simulink model "feedbacklin"  (R2020b)
settings: Solver=VariableStepAuto  StartTime=0.0  StopTime=40  RelTol=1e-3
values from neighbouring files (symbols this model uses):
  Ax = 25    [main.m]
  Ay = 25    [main.m]
  d2x = sym('d2x', 'real')    [AL.m]    (also in FL.m; main.m = 0)
  d2z = sym('d2z', 'real')    [AL.m]    (also in FL.m; main.m = 0.0979)
  dgx = sym('dgx', 'real')    [AL.m]    (also in FL.m; main.m = 0)
  gravity = sym('gravity','real')    [AL.m]    (also in FL.m; main.m = 9.81)
  J1 = sym('J1', 'real')    [AL.m]    (also in FL.m; main.m = 0.0154)
  J2 = sym('J2', 'real')    [AL.m]    (also in FL.m; main.m = 0.0011)
  Jm = sym('Jm', 'real')    [AL.m]    (also in FL.m; main.m = 0.4101)
  m1 = sym('m1','real')    [AL.m]    (also in FL.m; main.m = 1.309)
  m2 = sym('m2','real')    [AL.m]    (also in FL.m; main.m = 0.098)
  mM = sym('mM','real')    [AL.m]    (also in FL.m = sym('m','real'); main.m = 0.06)
  selector = select(1)    [main.m]    (also in select.m = input('? '))
  wx = 0.16    [main.m]
  wy = 0.16    [main.m]
(part 1 of 2)
settings Model: Creator=Tommaso  LastModifiedBy=Tommaso
settings DataIOCC: ReturnWorkspaceOutputs=off

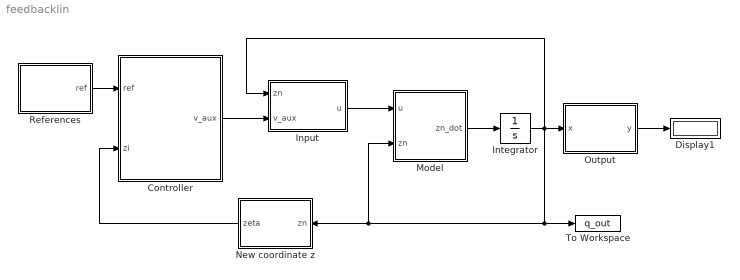
== system feedbacklin ==
  Controller : MATLAB Function  TreatAsAtomicUnit=on
  Display1 : Display
  Input : MATLAB Function  TreatAsAtomicUnit=on
  Integrator : Integrator  InitialCondition=[0; 0; 0; 0; 0; 0; 0; 0; (m1+m2+mM)*gravity; 0; 0; 0]
  Model : MATLAB Function  TreatAsAtomicUnit=on
  New coordinate z : MATLAB Function  TreatAsAtomicUnit=on
  Output : MATLAB Function  TreatAsAtomicUnit=on
  References : Subsystem
  To Workspace : ToWorkspace  VariableName=q_out  SaveFormat=Timeseries  SampleTime=-1
  wires:
  Output/1(y) -> Display1/1
  Integrator/1 -> Output/1(x), To Workspace/1, Model/2(zn), New coordinate z/1(zn), Input/1(zn)
  Model/1(zn_dot) -> Integrator/1
  Input/1(u) -> Model/1(u)
  Controller/1(v_aux) -> Input/2(v_aux)
  New coordinate z/1(zeta) -> Controller/2(zi)
  References/1(ref) -> Controller/1(ref)

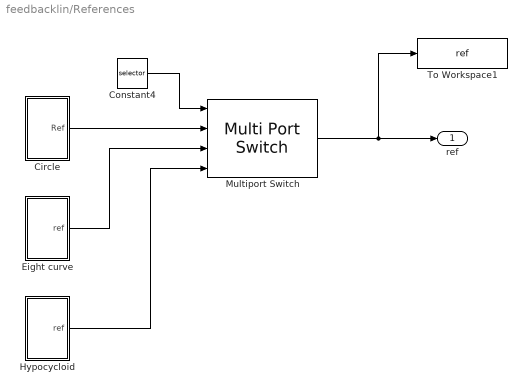
== system feedbacklin/References ==
  Circle : Subsystem
  Constant4 : Constant  Value=selector
  Eight curve : Subsystem
  Hypocycloid : Subsystem
  Multiport Switch : MultiPortSwitch
  To Workspace1 : ToWorkspace  VariableName=ref  SaveFormat=Timeseries  SampleTime=-1
  ref : Outport
  wires:
  Multiport Switch/1 -> To Workspace1/1, ref/1
  Constant4/1 -> Multiport Switch/1
  Eight curve/1(ref) -> Multiport Switch/3
  Circle/1(Ref) -> Multiport Switch/2
  Hypocycloid/1(ref) -> Multiport Switch/4

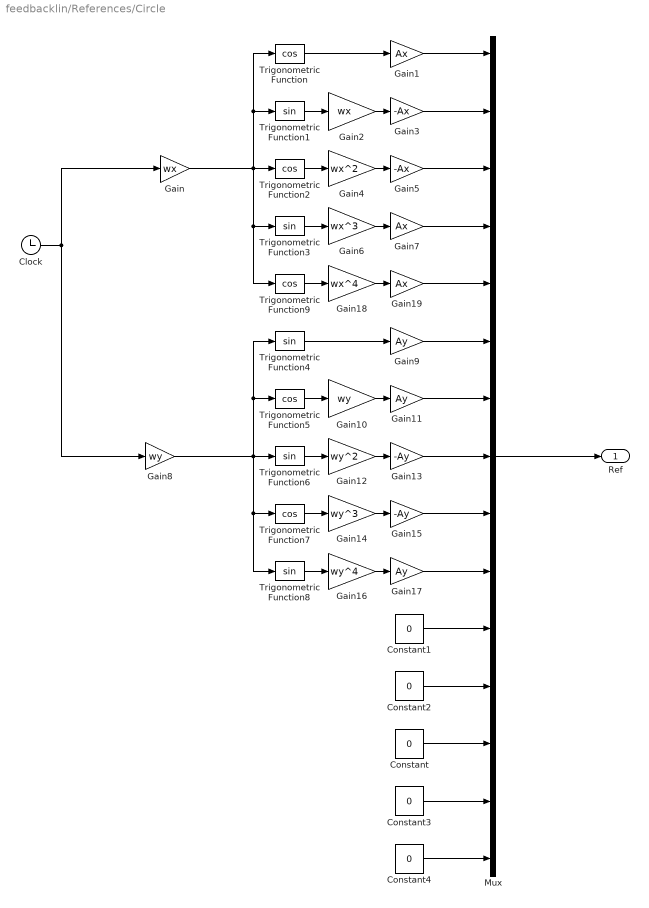
== system feedbacklin/References/Circle ==
  Clock : Clock
  Constant{,1..4} (5 alike) : Constant  Value=0
  Gain : Gain  Gain=wx
  Gain1 : Gain  Gain=Ax
  Gain10 : Gain  Gain=wy
  Gain11 : Gain  Gain=Ay
  Gain12 : Gain  Gain=wy^2
  Gain13 : Gain  Gain=-Ay
  Gain14 : Gain  Gain=wy^3
  Gain15 : Gain  Gain=-Ay
  Gain16 : Gain  Gain=wy^4
  Gain17 : Gain  Gain=Ay
  Gain18 : Gain  Gain=wx^4
  Gain19 : Gain  Gain=Ax
  Gain2 : Gain  Gain=wx
  Gain3 : Gain  Gain=-Ax
  Gain4 : Gain  Gain=wx^2
  Gain5 : Gain  Gain=-Ax
  Gain6 : Gain  Gain=wx^3
  Gain7 : Gain  Gain=Ax
  Gain8 : Gain  Gain=wy
  Gain9 : Gain  Gain=Ay
  Mux : Mux  Inputs=15
  Trigonometric Function{,2,5,7,9} (5 alike) : Trigonometry  Operator=cos
  Trigonometric Function{1,3..4,6,8} (5 alike) : Trigonometry
  Ref : Outport
  wires:
  Gain11/1 -> Mux/7
  Gain8/1 -> Trigonometric Function4/1, Trigonometric Function5/1, Trigonometric Function6/1, Trigonometric Function8/1, Trigonometric Function7/1
  Gain13/1 -> Mux/8
  Gain7/1 -> Mux/4
  Constant/1 -> Mux/13
  Constant3/1 -> Mux/14
  Gain6/1 -> Gain7/1
  Trigonometric Function5/1 -> Gain10/1
  Trigonometric Function3/1 -> Gain6/1
  Gain/1 -> Trigonometric Function/1, Trigonometric Function1/1, Trigonometric Function9/1, Trigonometric Function3/1, Trigonometric Function2/1
  Constant2/1 -> Mux/12
  Trigonometric Function2/1 -> Gain4/1
  Gain15/1 -> Mux/9
  Gain10/1 -> Gain11/1
  Gain5/1 -> Mux/3
  Gain2/1 -> Gain3/1
  Clock/1 -> Gain/1, Gain8/1
  Gain19/1 -> Mux/5
  Trigonometric Function6/1 -> Gain12/1
  Gain4/1 -> Gain5/1
  Constant4/1 -> Mux/15
  Trigonometric Function1/1 -> Gain2/1
  Gain12/1 -> Gain13/1
  Trigonometric Function9/1 -> Gain18/1
  Trigonometric Function/1 -> Gain1/1
  Trigonometric Function4/1 -> Gain9/1
  Gain17/1 -> Mux/10
  Trigonometric Function8/1 -> Gain16/1
  Gain1/1 -> Mux/1
  Mux/1 -> Ref/1
  Gain9/1 -> Mux/6
  Gain16/1 -> Gain17/1
  Gain14/1 -> Gain15/1
  Gain18/1 -> Gain19/1
  Constant1/1 -> Mux/11
  Gain3/1 -> Mux/2
  Trigonometric Function7/1 -> Gain14/1

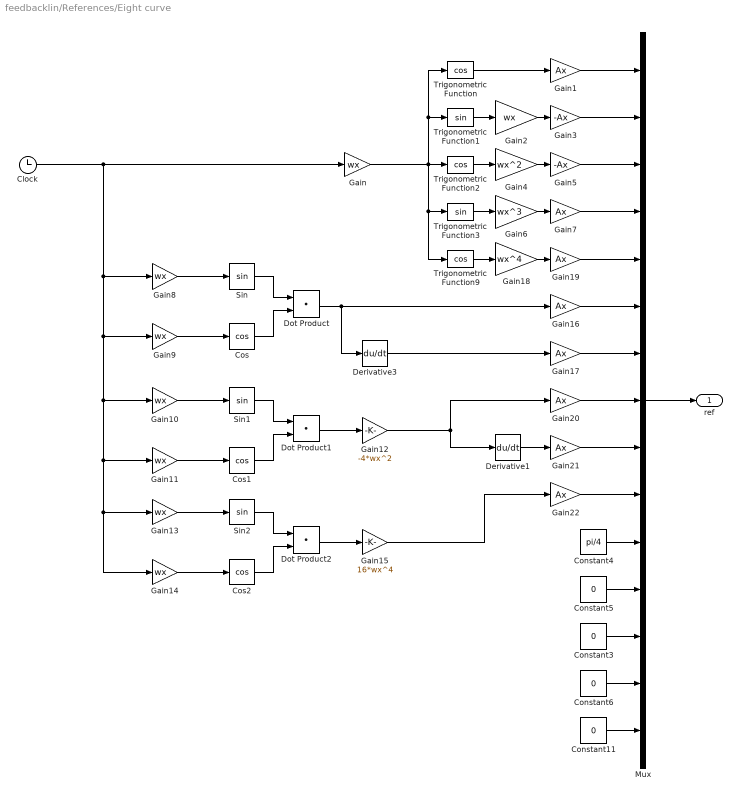
== system feedbacklin/References/Eight curve ==
  Clock : Clock
  Constant{3,5..6,11} (4 alike) : Constant  Value=0
  Constant4 : Constant  Value=pi/4
  Cos : Trigonometry  Operator=cos
  Cos1 : Trigonometry  Operator=cos
  Cos2 : Trigonometry  Operator=cos
  Derivative1 : Derivative
  Derivative3 : Derivative
  Dot Product : DotProduct  InputSameDT=on  OutDataTypeStr=Inherit: Inherit via internal rule
  Dot Product1 : DotProduct  InputSameDT=on  OutDataTypeStr=Inherit: Inherit via internal rule
  Dot Product2 : DotProduct  InputSameDT=on  OutDataTypeStr=Inherit: Inherit via internal rule
  Gain{,2,8..11,13..14} (8 alike) : Gain  Gain=wx
  Gain{1,7,16..17,19..22} (8 alike) : Gain  Gain=Ax
  Gain12 : Gain  Gain=-4*wx^2
  Gain15 : Gain  Gain=16*wx^4
  Gain18 : Gain  Gain=wx^4
  Gain3 : Gain  Gain=-Ax
  Gain4 : Gain  Gain=wx^2
  Gain5 : Gain  Gain=-Ax
  Gain6 : Gain  Gain=wx^3
  Mux : Mux  Inputs=15
  Sin : Trigonometry
  Sin1 : Trigonometry
  Sin2 : Trigonometry
  Trigonometric Function : Trigonometry  Operator=cos
  Trigonometric Function1 : Trigonometry
  Trigonometric Function2 : Trigonometry  Operator=cos
  Trigonometric Function3 : Trigonometry
  Trigonometric Function9 : Trigonometry  Operator=cos
  ref : Outport
  wires:
  Mux/1 -> ref/1
  Constant5/1 -> Mux/12
  Constant3/1 -> Mux/13
  Constant6/1 -> Mux/14
  Constant4/1 -> Mux/11
  Constant11/1 -> Mux/15
  Trigonometric Function1/1 -> Gain2/1
  Gain4/1 -> Gain5/1
  Gain5/1 -> Mux/3
  Trigonometric Function/1 -> Gain1/1
  Gain7/1 -> Mux/4
  Gain/1 -> Trigonometric Function9/1, Trigonometric Function3/1, Trigonometric Function/1, Trigonometric Function1/1, Trigonometric Function2/1
  Trigonometric Function2/1 -> Gain4/1
  Gain18/1 -> Gain19/1
  Trigonometric Function9/1 -> Gain18/1
  Gain3/1 -> Mux/2
  Trigonometric Function3/1 -> Gain6/1
  Gain19/1 -> Mux/5
  Gain6/1 -> Gain7/1
  Gain2/1 -> Gain3/1
  Gain1/1 -> Mux/1
  Derivative1/1 -> Gain21/1
  Derivative3/1 -> Gain17/1
  Dot Product/1 -> Derivative3/1, Gain16/1
  Sin/1 -> Dot Product/1
  Cos/1 -> Dot Product/2
  Gain9/1 -> Cos/1
  Gain8/1 -> Sin/1
  Gain10/1 -> Sin1/1
  Sin1/1 -> Dot Product1/1
  Gain11/1 -> Cos1/1
  Cos1/1 -> Dot Product1/2
  Dot Product1/1 -> Gain12/1
  Gain12/1 -> Derivative1/1, Gain20/1
  Dot Product2/1 -> Gain15/1
  Cos2/1 -> Dot Product2/2
  Sin2/1 -> Dot Product2/1
  Clock/1 -> Gain14/1, Gain13/1, Gain11/1, Gain10/1, Gain9/1, Gain8/1, Gain/1
  Gain14/1 -> Cos2/1
  Gain13/1 -> Sin2/1
  Gain15/1 -> Gain22/1
  Gain16/1 -> Mux/6
  Gain17/1 -> Mux/7
  Gain20/1 -> Mux/8
  Gain21/1 -> Mux/9
  Gain22/1 -> Mux/10

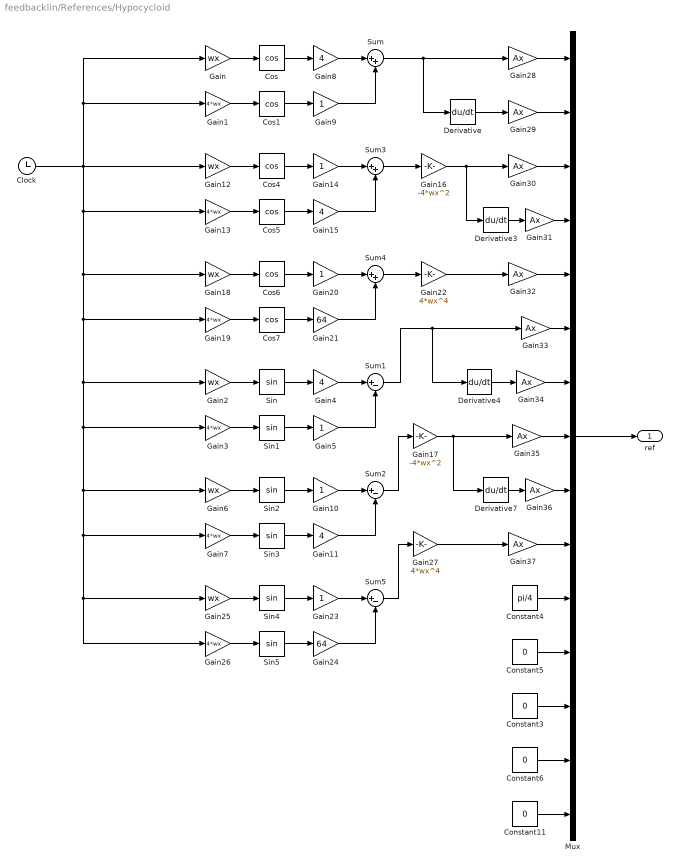
== system feedbacklin/References/Hypocycloid ==
  Clock : Clock
  Constant{3,5..6,11} (4 alike) : Constant  Value=0
  Constant4 : Constant  Value=pi/4
  Cos{,1,4..7} (6 alike) : Trigonometry  Operator=cos
  Derivative{,3..4,7} (4 alike) : Derivative
  Gain{,2,6,12,18,25} (6 alike) : Gain  Gain=wx
  Gain{1,3,7,13,19,26} (6 alike) : Gain  Gain=4*wx
  Gain{5,9..10,14,20,23} (6 alike) : Gain
  Gain{4,8,11,15} (4 alike) : Gain  Gain=4
  Gain16 : Gain  Gain=-4*wx^2
  Gain17 : Gain  Gain=-4*wx^2
  Gain21 : Gain  Gain=64
  Gain22 : Gain  Gain=4*wx^4
  Gain24 : Gain  Gain=64
  Gain27 : Gain  Gain=4*wx^4
  Gain{28..37} (10 alike) : Gain  Gain=Ax
  Mux : Mux  Inputs=15
  Sin{,1..5} (6 alike) : Trigonometry
  Sum : Sum  Inputs=|++
  Sum1 : Sum  Inputs=|+-
  Sum2 : Sum  Inputs=|+-
  Sum3 : Sum  Inputs=|++
  Sum4 : Sum  Inputs=|++
  Sum5 : Sum  Inputs=|+-
  ref : Outport
  wires:
  Mux/1 -> ref/1
  Constant5/1 -> Mux/12
  Constant3/1 -> Mux/13
  Constant6/1 -> Mux/14
  Constant4/1 -> Mux/11
  Constant11/1 -> Mux/15
  Cos/1 -> Gain8/1
  Gain8/1 -> Sum/1
  Cos1/1 -> Gain9/1
  Gain9/1 -> Sum/2
  Sum/1 -> Gain28/1, Derivative/1
  Gain/1 -> Cos/1
  Gain1/1 -> Cos1/1
  Sin1/1 -> Gain5/1
  Gain4/1 -> Sum1/1
  Sin/1 -> Gain4/1
  Gain3/1 -> Sin1/1
  Gain5/1 -> Sum1/2
  Gain2/1 -> Sin/1
  Sum1/1 -> Gain33/1, Derivative4/1
  Derivative4/1 -> Gain34/1
  Sum2/1 -> Gain17/1
  Gain17/1 -> Gain35/1, Derivative7/1
  Gain13/1 -> Cos5/1
  Gain12/1 -> Cos4/1
  Gain15/1 -> Sum3/2
  Cos4/1 -> Gain14/1
  Gain14/1 -> Sum3/1
  Cos5/1 -> Gain15/1
  Sum3/1 -> Gain16/1
  Derivative3/1 -> Gain31/1
  Gain16/1 -> Derivative3/1, Gain30/1
  Gain21/1 -> Sum4/2
  Cos7/1 -> Gain21/1
  Cos6/1 -> Gain20/1
  Gain18/1 -> Cos6/1
  Gain19/1 -> Cos7/1
  Sum4/1 -> Gain22/1
  Gain20/1 -> Sum4/1
  Gain22/1 -> Gain32/1
  Derivative7/1 -> Gain36/1
  Gain10/1 -> Sum2/1
  Gain7/1 -> Sin3/1
  Sin3/1 -> Gain11/1
  Sin2/1 -> Gain10/1
  Gain6/1 -> Sin2/1
  Gain11/1 -> Sum2/2
  Gain24/1 -> Sum5/2
  Gain26/1 -> Sin5/1
  Gain23/1 -> Sum5/1
  Sin4/1 -> Gain23/1
  Gain25/1 -> Sin4/1
  Sum5/1 -> Gain27/1
  Clock/1 -> Gain1/1, Gain/1, Gain12/1, Gain13/1, Gain26/1, Gain25/1, Gain7/1, Gain6/1, Gain3/1, Gain2/1, Gain19/1, Gain18/1
  Sin5/1 -> Gain24/1
  Gain27/1 -> Gain37/1
  Gain28/1 -> Mux/1
  Derivative/1 -> Gain29/1
  Gain29/1 -> Mux/2
  Gain30/1 -> Mux/3
  Gain31/1 -> Mux/4
  Gain32/1 -> Mux/5
  Gain33/1 -> Mux/6
  Gain34/1 -> Mux/7
  Gain35/1 -> Mux/8
  Gain36/1 -> Mux/9
  Gain37/1 -> Mux/10

== matlab function feedbacklin/Model ==
  data: u input; zn input; zn_dot output; m1 parameter; m2 parameter; mM parameter; J1 parameter; J2 parameter; Jm parameter; d2x parameter; d2z parameter; dgx parameter; gravity parameter
function zn_dot = model(u, zn, m1, m2, mM, J1, J2, Jm, d2x, d2z, dgx, gravity)

% State variables
pc1x = zn(1);
pc1z = zn(2);
pc1x_dot = zn(3);
pc1z_dot = zn(4);
theta1 = zn(5);
theta1_dot = zn(6);
theta12 = zn(7);
theta12_dot = zn(8);
ut = zn(9);
tau = zn(10);
w1 = zn(11);
w2 = zn(12);

% Parameters
d2 = [d2x; d2z];
beta1 = -m2*(d2x*cos(theta12) + d2z*sin(theta12));
beta2 = -m2*(d2z*cos(theta12) - d2x*sin(theta12));
g4 = m2*gravity*(d2x*cos(theta12) + d2z*sin(theta12));
mb = J2 + Jm + m2*norm(d2)^2;
ms = m1 + m2 + mM;

% Dynamic matrices
g = [0; -ms*gravity; 0; g4];
C = [beta1*theta12_dot^2; beta2*theta12_dot^2; 0; 0];
M = [ms 0 0 beta1; 0 ms 0 beta2; 0 0 J1 0; beta1 beta2 0 mb];
G = [-sin(theta1) 0 0; -cos(theta1) 0 0; dgx 1 -1; 0 0 1];

% State vector (8x1):
x = [pc1x, pc1z, pc1x_dot, pc1z_dot, theta1, theta1_dot, theta12, theta12_dot]'; 

% Control field (8x3)
invMG = (M\G);
g_x = [0 0 0; 0 0 0; invMG(1,:); invMG(2,:); 0 0 0; invMG(3,:); 0 0 0; invMG(4,:)];

% New vector state (10x1)
z = [x; ut; tau];

% Control field (10x1)
g_z = [g_x(:,2); 0; 0];

% New vector state (12x1)
zn = [z; w1; w2];

% New state space representation
z1n_dot = zn(3);
z2n_dot = zn(4);
z5n_dot = zn(6);
z7n_dot = zn(8);

% We modify q_ddot because ut and tau are new states
q_new_ddot = (M\(G(:,1)*zn(9) + G(:,3)*zn(10) -C - g));

w1n = u(1);
w2n = u(3);
wn = [w1n; w2n];

z3n_dot = q_new_ddot(1);
z4n_dot = q_new_ddot(2);
z6n_dot = q_new_ddot(3);
z8n_dot = q_new_ddot(4);
z9n_dot = w1;
z10n_dot = w2;

% Drift field (12x1)
fn_z = [z1n_dot; z2n_dot; z3n_dot; z4n_dot; z5n_dot; z6n_dot; z7n_dot; z8n_dot; z9n_dot; z10n_dot; 0; 0];

% Control field (12x1)
gn_z = [g_z; 0; 0];
gn_w = [0 0; 0 0; 0 0; 0 0; 0 0; 0 0; 0 0; 0 0 ; 0 0; 0 0; 1 0; 0 1];

% New Affine-form system
zn_dot = fn_z + gn_z*u(2) + gn_w*wn;

== matlab function feedbacklin/Input ==
  data: zn input; u output; v_aux input; m1 parameter; m2 parameter; mM parameter; J1 parameter; J2 parameter; Jm parameter; d2x parameter; d2z parameter; dgx parameter; gravity parameter
function u = input(zn, v_aux,m1, m2, mM, J1, J2, Jm, d2x, d2z, dgx, gravity)

% State variables
theta1 = zn(5);
theta1_dot = zn(6);
theta12 = zn(7);
theta12_dot = zn(8);
ut = zn(9);
tau = zn(10);
w1 = zn(11);
w2 = zn(12);

% Parameters
d2 = [d2x; d2z];
mb = J2 + Jm + m2*norm(d2)^2;
ms = m1 + m2 + mM;

% Gamma (3x1)
gamma = [(((m2*(d2z^2*m2*ut*cos(theta1 - 2*theta12) - d2x^2*m2*ut*cos(theta1 - 2*theta12) - d2z*ms*tau*cos(theta12) + d2x*ms*tau*sin(theta12) + 2*d2x*d2z*m2*ut*sin(theta1 - 2*theta12) - d2z*mb*ms*theta12_dot^2*cos(theta12) + d2x*mb*ms*theta12_dot^2*sin(theta12) + d2x^2*gravity*m2*ms*cos(2*theta12) - d2z^2*gravity*m2*ms*cos(2*theta12) - d2x^2*gravity*m2*ms*sin(2*theta12) + d2z^2*gravity*m2*ms*sin(2*theta12) + 2*d2x*d2z*gravity*m2*ms*cos(2*theta12) + 2*d2x*d2z*gravity*m2*ms*sin(2*theta12)))/(ms*(d2x^2*m2^2 + d2z^2*m2^2 - mb*ms)) - (2*m2*mb*theta12_dot^2*(d2z*cos(theta12) - d2x*sin(theta12)))/(d2x^2*m2^2 + d2z^2*m2^2 - mb*ms) - (2*m2*mb*(d2x*cos(theta12) + d2z*sin(theta12))*(d2z*m2*ut*cos(theta1 - theta12) - d2x^2*m2^2*theta12_dot^2 - d2z^2*m2^2*theta12_dot^2 - ms*tau + d2x*m2*ut*sin(theta1 - theta12) + d2x*gravity*m2*ms*cos(theta12) - d2z*gravity*m2*ms*cos(theta12) + d2x*gravity*m2*ms*sin(theta12) + d2z*gravity*m2*ms*sin(theta12)))/(d2x^2*m2^2 + d2z^2*m2^2 - mb*ms)^2 + (4*m2^3*mb*theta12_dot^2*(d2x*cos(theta12) + d2z*sin(theta12))*(d2x^2 + d2z^2))/(d2x^2*m2^2 + d2z^2*m2^2 - mb*ms)^2)*(d2z*m2*ut*cos(theta1 - theta12) - d2x^2*m2^2*theta12_dot^2 - d2z^2*m2^2*theta12_dot^2 - ms*tau + d2x*m2*ut*sin(theta1 - theta12) + d2x*gravity*m2*ms*cos(theta12) - d2z*gravity*m2*ms*cos(theta12) + d2x*gravity*m2*ms*sin(theta12) + d2z*gravity*m2*ms*sin(theta12)))/(d2x^2*m2^2 + d2z^2*m2^2 - mb*ms) - w2*((m2*theta12_dot*(d2z*cos(theta12) - d2x*sin(theta12)))/(d2x^2*m2^2 + d2z^2*m2^2 - mb*ms) - (2*m2*mb*ms*theta12_dot*(d2x*cos(theta12) + d2z*sin(theta12)))/(d2x^2*m2^2 + d2z^2*m2^2 - mb*ms)^2) - theta1_dot*((w1*(d2x^2*m2^2*cos(theta1) - 2*mb*ms*cos(theta1) + d2z^2*m2^2*cos(theta1) - d2x^2*m2^2*cos(theta1 - 2*theta12) + d2z^2*m2^2*cos(theta1 - 2*theta12) + 2*d2x*d2z*m2^2*sin(theta1 - 2*theta12)))/(2*ms*(d2x^2*m2^2 + d2z^2*m2^2 - mb*ms)) + (theta1_dot*ut*(d2x^2*m2^2*sin(theta1 - 2*theta12) - d2z^2*m2^2*sin(theta1 - 2*theta12) + 2*mb*ms*sin(theta1) - d2x^2*m2^2*sin(theta1) - d2z^2*m2^2*sin(theta1) + 2*d2x*d2z*m2^2*cos(theta1 - 2*theta12)))/(2*ms*(d2x^2*m2^2 + d2z^2*m2^2 - mb*ms)) - (m2^2*theta12_dot*ut*(sin(theta1 - 2*theta12)*d2x^2 + 2*cos(theta1 - 2*theta12)*d2x*d2z - sin(theta1 - 2*theta12)*d2z^2))/(ms*(d2x^2*m2^2 + d2z^2*m2^2 - mb*ms)) + (2*m2^2*mb*theta12_dot*ut*(d2x*cos(theta1 - theta12) - d2z*sin(theta1 - theta12))*(d2x*cos(theta12) + d2z*sin(theta12)))/(d2x^2*m2^2 + d2z^2*m2^2 - mb*ms)^2) - theta12_dot*((m2*w2*(d2z*cos(theta12) - d2x*sin(theta12)))/(d2x^2*m2^2 + d2z^2*m2^2 - mb*ms) - (m2*theta12_dot*(2*d2z^2*m2*ut*sin(theta1 - 2*theta12) - 2*d2x^2*m2*ut*sin(theta1 - 2*theta12) + d2x*ms*tau*cos(theta12) + d2z*ms*tau*sin(theta12) - 4*d2x*d2z*m2*ut*cos(theta1 - 2*theta12) + d2x*mb*ms*theta12_dot^2*cos(theta12) + d2z*mb*ms*theta12_dot^2*sin(theta12) - 2*d2x^2*gravity*m2*ms*cos(2*theta12) + 2*d2z^2*gravity*m2*ms*cos(2*theta12) - 2*d2x^2*gravity*m2*ms*sin(2*theta12) + 2*d2z^2*gravity*m2*ms*sin(2*theta12) + 4*d2x*d2z*gravity*m2*ms*cos(2*theta12) - 4*d2x*d2z*gravity*m2*ms*sin(2*theta12)))/(ms*(d2x^2*m2^2 + d2z^2*m2^2 - mb*ms)) - (m2^2*w1*(- cos(theta1 - 2*theta12)*d2x^2 + 2*sin(theta1 - 2*theta12)*d2x*d2z + cos(theta1 - 2*theta12)*d2z^2))/(ms*(d2x^2*m2^2 + d2z^2*m2^2 - mb*ms)) + (2*m2*mb*theta12_dot*(d2z*cos(theta12) - d2x*sin(theta12))*(d2z*m2*ut*cos(theta1 - theta12) - d2x^2*m2^2*theta12_dot^2 - d2z^2*m2^2*theta12_dot^2 - ms*tau + d2x*m2*ut*sin(theta1 - theta12) + d2x*gravity*m2*ms*cos(theta12) - d2z*gravity*m2*ms*cos(theta12) + d2x*gravity*m2*ms*sin(theta12) + d2z*gravity*m2*ms*sin(theta12)))/(d2x^2*m2^2 + d2z^2*m2^2 - mb*ms)^2 + (2*m2^2*mb*theta12_dot*(d2x*cos(theta12) + d2z*sin(theta12))*(d2z*ut*sin(theta1 - theta12) - d2x*ut*cos(theta1 - theta12) + d2x*gravity*ms*cos(theta12) + d2z*gravity*ms*cos(theta12) - d2x*gravity*ms*sin(theta12) + d2z*gravity*ms*sin(theta12)))/(d2x^2*m2^2 + d2z^2*m2^2 - mb*ms)^2 - (m2^2*theta1_dot*ut*(sin(theta1 - 2*theta12)*d2x^2 + 2*cos(theta1 - 2*theta12)*d2x*d2z - sin(theta1 - 2*theta12)*d2z^2))/(ms*(d2x^2*m2^2 + d2z^2*m2^2 - mb*ms))) - w1*((theta1_dot*(d2x^2*m2^2*cos(theta1) - 2*mb*ms*cos(theta1) + d2z^2*m2^2*cos(theta1) - d2x^2*m2^2*cos(theta1 - 2*theta12) + d2z^2*m2^2*cos(theta1 - 2*theta12) + 2*d2x*d2z*m2^2*sin(theta1 - 2*theta12)))/(2*ms*(d2x^2*m2^2 + d2z^2*m2^2 - mb*ms)) - (m2^2*theta12_dot*(- cos(theta1 - 2*theta12)*d2x^2 + 2*sin(theta1 - 2*theta12)*d2x*d2z + cos(theta1 - 2*theta12)*d2z^2))/(ms*(d2x^2*m2^2 + d2z^2*m2^2 - mb*ms)) + (2*m2^2*mb*theta12_dot*(d2z*cos(theta1 - theta12) + d2x*sin(theta1 - theta12))*(d2x*cos(theta12) + d2z*sin(theta12)))/(d2x^2*m2^2 + d2z^2*m2^2 - mb*ms)^2) + (ut*(tau - dgx*ut)*(d2x^2*m2^2*cos(theta1) - 2*mb*ms*cos(theta1) + d2z^2*m2^2*cos(theta1) - d2x^2*m2^2*cos(theta1 - 2*theta12) + d2z^2*m2^2*cos(theta1 - 2*theta12) + 2*d2x*d2z*m2^2*sin(theta1 - 2*theta12)))/(2*J1*ms*(d2x^2*m2^2 + d2z^2*m2^2 - mb*ms))
             w2*((m2*theta12_dot*(d2x*cos(theta12) + d2z*sin(theta12)))/(d2x^2*m2^2 + d2z^2*m2^2 - mb*ms) + (2*m2*mb*ms*theta12_dot*(d2z*cos(theta12) - d2x*sin(theta12)))/(d2x^2*m2^2 + d2z^2*m2^2 - mb*ms)^2) + theta1_dot*((w1*(d2x^2*m2^2*sin(theta1 - 2*theta12) - d2z^2*m2^2*sin(theta1 - 2*theta12) - 2*mb*ms*sin(theta1) + d2x^2*m2^2*sin(theta1) + d2z^2*m2^2*sin(theta1) + 2*d2x*d2z*m2^2*cos(theta1 - 2*theta12)))/(2*ms*(d2x^2*m2^2 + d2z^2*m2^2 - mb*ms)) - (theta1_dot*ut*(2*mb*ms*cos(theta1) - d2x^2*m2^2*cos(theta1) - d2z^2*m2^2*cos(theta1) - d2x^2*m2^2*cos(theta1 - 2*theta12) + d2z^2*m2^2*cos(theta1 - 2*theta12) + 2*d2x*d2z*m2^2*sin(theta1 - 2*theta12)))/(2*ms*(d2x^2*m2^2 + d2z^2*m2^2 - mb*ms)) + (m2^2*theta12_dot*ut*(- cos(theta1 - 2*theta12)*d2x^2 + 2*sin(theta1 - 2*theta12)*d2x*d2z + cos(theta1 - 2*theta12)*d2z^2))/(ms*(d2x^2*m2^2 + d2z^2*m2^2 - mb*ms)) - (2*m2^2*mb*theta12_dot*ut*(d2x*cos(theta1 - theta12) - d2z*sin(theta1 - theta12))*(d2z*cos(theta12) - d2x*sin(theta12)))/(d2x^2*m2^2 + d2z^2*m2^2 - mb*ms)^2) + theta12_dot*((m2*w2*(d2x*cos(theta12) + d2z*sin(theta12)))/(d2x^2*m2^2 + d2z^2*m2^2 - mb*ms) - (m2*theta12_dot*(2*d2z^2*m2*ut*cos(theta1 - 2*theta12) - 2*d2x^2*m2*ut*cos(theta1 - 2*theta12) - d2z*ms*tau*cos(theta12) + d2x*ms*tau*sin(theta12) + 4*d2x*d2z*m2*ut*sin(theta1 - 2*theta12) - d2z*mb*ms*theta12_dot^2*cos(theta12) + d2x*mb*ms*theta12_dot^2*sin(theta12) + 2*d2x^2*gravity*m2*ms*cos(2*theta12) - 2*d2z^2*gravity*m2*ms*cos(2*theta12) - 2*d2x^2*gravity*m2*ms*sin(2*theta12) + 2*d2z^2*gravity*m2*ms*sin(2*theta12) + 4*d2x*d2z*gravity*m2*ms*cos(2*theta12) + 4*d2x*d2z*gravity*m2*ms*sin(2*theta12)))/(ms*(d2x^2*m2^2 + d2z^2*m2^2 - mb*ms)) - (m2^2*w1*(sin(theta1 - 2*theta12)*d2x^2 + 2*cos(theta1 - 2*theta12)*d2x*d2z - sin(theta1 - 2*theta12)*d2z^2))/(ms*(d2x^2*m2^2 + d2z^2*m2^2 - mb*ms)) + (2*m2*mb*theta12_dot*(d2x*cos(theta12) + d2z*sin(theta12))*(d2z*m2*ut*cos(theta1 - theta12) - d2x^2*m2^2*theta12_dot^2 - d2z^2*m2^2*theta12_dot^2 - ms*tau + d2x*m2*ut*sin(theta1 - theta12) + d2x*gravity*m2*ms*cos(theta12) - d2z*gravity*m2*ms*cos(theta12) + d2x*gravity*m2*ms*sin(theta12) + d2z*gravity*m2*ms*sin(theta12)))/(d2x^2*m2^2 + d2z^2*m2^2 - mb*ms)^2 - (2*m2^2*mb*theta12_dot*(d2z*cos(theta12) - d2x*sin(theta12))*(d2z*ut*sin(theta1 - theta12) - d2x*ut*cos(theta1 - theta12) + d2x*gravity*ms*cos(theta12) + d2z*gravity*ms*cos(theta12) - d2x*gravity*ms*sin(theta12) + d2z*gravity*ms*sin(theta12)))/(d2x^2*m2^2 + d2z^2*m2^2 - mb*ms)^2 + (m2^2*theta1_dot*ut*(- cos(theta1 - 2*theta12)*d2x^2 + 2*sin(theta1 - 2*theta12)*d2x*d2z + cos(theta1 - 2*theta12)*d2z^2))/(ms*(d2x^2*m2^2 + d2z^2*m2^2 - mb*ms))) - w1*((m2^2*theta12_dot*(sin(theta1 - 2*theta12)*d2x^2 + 2*cos(theta1 - 2*theta12)*d2x*d2z - sin(theta1 - 2*theta12)*d2z^2))/(ms*(d2x^2*m2^2 + d2z^2*m2^2 - mb*ms)) - (theta1_dot*(d2x^2*m2^2*sin(theta1 - 2*theta12) - d2z^2*m2^2*sin(theta1 - 2*theta12) - 2*mb*ms*sin(theta1) + d2x^2*m2^2*sin(theta1) + d2z^2*m2^2*sin(theta1) + 2*d2x*d2z*m2^2*cos(theta1 - 2*theta12)))/(2*ms*(d2x^2*m2^2 + d2z^2*m2^2 - mb*ms)) + (2*m2^2*mb*theta12_dot*(d2z*cos(theta1 - theta12) + d2x*sin(theta1 - theta12))*(d2z*cos(theta12) - d2x*sin(theta12)))/(d2x^2*m2^2 + d2z^2*m2^2 - mb*ms)^2) + (((m2*(d2z^2*m2*ut*sin(theta1 - 2*theta12) - d2x^2*m2*ut*sin(theta1 - 2*theta12) + d2x*ms*tau*cos(theta12) + d2z*ms*tau*sin(theta12) - 2*d2x*d2z*m2*ut*cos(theta1 - 2*theta12) + d2x*mb*ms*theta12_dot^2*cos(theta12) + d2z*mb*ms*theta12_dot^2*sin(theta12) - d2x^2*gravity*m2*ms*cos(2*theta12) + d2z^2*gravity*m2*ms*cos(2*theta12) - d2x^2*gravity*m2*ms*sin(2*theta12) + d2z^2*gravity*m2*ms*sin(2*theta12) + 2*d2x*d2z*gravity*m2*ms*cos(2*theta12) - 2*d2x*d2z*gravity*m2*ms*sin(2*theta12)))/(ms*(d2x^2*m2^2 + d2z^2*m2^2 - mb*ms)) + (2*m2*mb*theta12_dot^2*(d2x*cos(theta12) + d2z*sin(theta12)))/(d2x^2*m2^2 + d2z^2*m2^2 - mb*ms) - (2*m2*mb*(d2z*cos(theta12) - d2x*sin(theta12))*(d2z*m2*ut*cos(theta1 - theta12) - d2x^2*m2^2*theta12_dot^2 - d2z^2*m2^2*theta12_dot^2 - ms*tau + d2x*m2*ut*sin(theta1 - theta12) + d2x*gravity*m2*ms*cos(theta12) - d2z*gravity*m2*ms*cos(theta12) + d2x*gravity*m2*ms*sin(theta12) + d2z*gravity*m2*ms*sin(theta12)))/(d2x^2*m2^2 + d2z^2*m2^2 - mb*ms)^2 + (4*m2^3*mb*theta12_dot^2*(d2z*cos(theta12) - d2x*sin(theta12))*(d2x^2 + d2z^2))/(d2x^2*m2^2 + d2z^2*m2^2 - mb*ms)^2)*(d2z*m2*ut*cos(theta1 - theta12) - d2x^2*m2^2*theta12_dot^2 - d2z^2*m2^2*theta12_dot^2 - ms*tau + d2x*m2*ut*sin(theta1 - theta12) + d2x*gravity*m2*ms*cos(theta12) - d2z*gravity*m2*ms*cos(theta12) + d2x*gravity*m2*ms*sin(theta12) + d2z*gravity*m2*ms*sin(theta12)))/(d2x^2*m2^2 + d2z^2*m2^2 - mb*ms) - (ut*(tau - dgx*ut)*(d2x^2*m2^2*sin(theta1 - 2*theta12) - d2z^2*m2^2*sin(theta1 - 2*theta12) - 2*mb*ms*sin(theta1) + d2x^2*m2^2*sin(theta1) + d2z^2*m2^2*sin(theta1) + 2*d2x*d2z*m2^2*cos(theta1 - 2*theta12)))/(2*J1*ms*(d2x^2*m2^2 + d2z^2*m2^2 - mb*ms))
                                                                                                                                                                                                                                                                                                                                                                                                                                                                                                                                                                                                                                                                                                                                                                                                                                                                                                                                                                                                                                                                                                                                                                                                                                                                                                                                                                                                                                                                                                                                                                                                                                                                                                                                                                                                                                                                                                                                                                                                                                                                                                                                                                                                                                          theta1_dot*((m2*w1*(d2x*cos(theta1 - theta12) - d2z*sin(theta1 - theta12)))/(d2x^2*m2^2 + d2z^2*m2^2 - mb*ms) - (m2*theta1_dot*ut*(d2z*cos(theta1 - theta12) + d2x*sin(theta1 - theta12)))/(d2x^2*m2^2 + d2z^2*m2^2 - mb*ms) + (m2*theta12_dot*ut*(d2z*cos(theta1 - theta12) + d2x*sin(theta1 - theta12)))/(d2x^2*m2^2 + d2z^2*m2^2 - mb*ms) - (2*m2^3*theta12_dot*ut*(d2x*cos(theta1 - theta12) - d2z*sin(theta1 - theta12))*(d2x^2 + d2z^2))/(d2x^2*m2^2 + d2z^2*m2^2 - mb*ms)^2) - theta12_dot*((m2*w1*(d2x*cos(theta1 - theta12) - d2z*sin(theta1 - theta12)))/(d2x^2*m2^2 + d2z^2*m2^2 - mb*ms) + (m2*theta12_dot*(d2z*ut*cos(theta1 - theta12) + d2x*ut*sin(theta1 - theta12) + d2x*gravity*ms*cos(theta12) - d2z*gravity*ms*cos(theta12) + d2x*gravity*ms*sin(theta12) + d2z*gravity*ms*sin(theta12)))/(d2x^2*m2^2 + d2z^2*m2^2 - mb*ms) + (2*m2^3*theta12_dot*(d2x^2 + d2z^2)*(d2z*ut*sin(theta1 - theta12) - d2x*ut*cos(theta1 - theta12) + d2x*gravity*ms*cos(theta12) + d2z*gravity*ms*cos(theta12) - d2x*gravity*ms*sin(theta12) + d2z*gravity*ms*sin(theta12)))/(d2x^2*m2^2 + d2z^2*m2^2 - mb*ms)^2 - (m2*theta1_dot*ut*(d2z*cos(theta1 - theta12) + d2x*sin(theta1 - theta12)))/(d2x^2*m2^2 + d2z^2*m2^2 - mb*ms)) - w1*((m2*theta12_dot*(d2x*cos(theta1 - theta12) - d2z*sin(theta1 - theta12)))/(d2x^2*m2^2 + d2z^2*m2^2 - mb*ms) - (m2*theta1_dot*(d2x*cos(theta1 - theta12) - d2z*sin(theta1 - theta12)))/(d2x^2*m2^2 + d2z^2*m2^2 - mb*ms) + (2*m2^3*theta12_dot*(d2z*cos(theta1 - theta12) + d2x*sin(theta1 - theta12))*(d2x^2 + d2z^2))/(d2x^2*m2^2 + d2z^2*m2^2 - mb*ms)^2) + (((m2*(d2z*ut*sin(theta1 - theta12) - d2x*ut*cos(theta1 - theta12) + d2x*gravity*ms*cos(theta12) + d2z*gravity*ms*cos(theta12) - d2x*gravity*ms*sin(theta12) + d2z*gravity*ms*sin(theta12)))/(d2x^2*m2^2 + d2z^2*m2^2 - mb*ms) - (2*m2^2*(d2x^2 + d2z^2)*(d2z*m2*ut*cos(theta1 - theta12) - d2x^2*m2^2*theta12_dot^2 - d2z^2*m2^2*theta12_dot^2 - ms*tau + d2x*m2*ut*sin(theta1 - theta12) + d2x*gravity*m2*ms*cos(theta12) - d2z*gravity*m2*ms*cos(theta12) + d2x*gravity*m2*ms*sin(theta12) + d2z*gravity*m2*ms*sin(theta12)))/(d2x^2*m2^2 + d2z^2*m2^2 - mb*ms)^2 + (4*m2^4*theta12_dot^2*(d2x^2 + d2z^2)^2)/(d2x^2*m2^2 + d2z^2*m2^2 - mb*ms)^2)*(d2z*m2*ut*cos(theta1 - theta12) - d2x^2*m2^2*theta12_dot^2 - d2z^2*m2^2*theta12_dot^2 - ms*tau + d2x*m2*ut*sin(theta1 - theta12) + d2x*gravity*m2*ms*cos(theta12) - d2z*gravity*m2*ms*cos(theta12) + d2x*gravity*m2*ms*sin(theta12) + d2z*gravity*m2*ms*sin(theta12)))/(d2x^2*m2^2 + d2z^2*m2^2 - mb*ms) + (2*m2^2*ms*theta12_dot*w2*(d2x^2 + d2z^2))/(d2x^2*m2^2 + d2z^2*m2^2 - mb*ms)^2 - (m2*ut*(d2x*cos(theta1 - theta12) - d2z*sin(theta1 - theta12))*(tau - dgx*ut))/(J1*(d2x^2*m2^2 + d2z^2*m2^2 - mb*ms))];
                                                                                                                                                                                                                                                                                                                                                                                                                                                                                                                                                                                                                                                                                                                                                                                                                                                                                                                                                                                                                                                                                                                                                                                                                                                                                                                                                                                                                                                                                                                                                                                                                                                                                                                                                                                                                                                                                                                                                                                                                                                                                                                                                                                                                                      

% E (3x3)                                                                                                                                                                                                                                                                                                                                                                                                                                                                                                                                                                                                                                                                                                                                                                                                                                                                                                                                                                                                                                                                                                                                                                                                                                                                                                                                                                                                                                                                                                                                                                                                                                                                                                                                                                                                                                                                                                                                                                                                                                                                                                                                                                                                                                    
E = [(d2x^2*m2^2*sin(theta1 - 2*theta12) - d2z^2*m2^2*sin(theta1 - 2*theta12) + 2*mb*ms*sin(theta1) - d2x^2*m2^2*sin(theta1) - d2z^2*m2^2*sin(theta1) + 2*d2x*d2z*m2^2*cos(theta1 - 2*theta12))/(2*ms*(d2x^2*m2^2 + d2z^2*m2^2 - mb*ms)), -(ut*(d2x^2*m2^2*cos(theta1) - 2*mb*ms*cos(theta1) + d2z^2*m2^2*cos(theta1) - d2x^2*m2^2*cos(theta1 - 2*theta12) + d2z^2*m2^2*cos(theta1 - 2*theta12) + 2*d2x*d2z*m2^2*sin(theta1 - 2*theta12)))/(2*J1*ms*(d2x^2*m2^2 + d2z^2*m2^2 - mb*ms)), -(m2*(d2x*cos(theta12) + d2z*sin(theta12)))/(d2x^2*m2^2 + d2z^2*m2^2 - mb*ms)
    (2*mb*ms*cos(theta1) - d2x^2*m2^2*cos(theta1) - d2z^2*m2^2*cos(theta1) - d2x^2*m2^2*cos(theta1 - 2*theta12) + d2z^2*m2^2*cos(theta1 - 2*theta12) + 2*d2x*d2z*m2^2*sin(theta1 - 2*theta12))/(2*ms*(d2x^2*m2^2 + d2z^2*m2^2 - mb*ms)),  (ut*(d2x^2*m2^2*sin(theta1 - 2*theta12) - d2z^2*m2^2*sin(theta1 - 2*theta12) - 2*mb*ms*sin(theta1) + d2x^2*m2^2*sin(theta1) + d2z^2*m2^2*sin(theta1) + 2*d2x*d2z*m2^2*cos(theta1 - 2*theta12)))/(2*J1*ms*(d2x^2*m2^2 + d2z^2*m2^2 - mb*ms)), -(m2*(d2z*cos(theta12) - d2x*sin(theta12)))/(d2x^2*m2^2 + d2z^2*m2^2 - mb*ms)
                                                                                                                                         (m2*(d2z*cos(theta1 - theta12) + d2x*sin(theta1 - theta12)))/(d2x^2*m2^2 + d2z^2*m2^2 - mb*ms),                                                                                                                                       (m2*ut*(d2x*cos(theta1 - theta12) - d2z*sin(theta1 - theta12)))/(J1*(d2x^2*m2^2 + d2z^2*m2^2 - mb*ms)),                                         -ms/(d2x^2*m2^2 + d2z^2*m2^2 - mb*ms)];
                                                                                                                                     
                                                                                                                                     
invE = inv(E);    
    
% Input (3x1)
u = invE*(v_aux - gamma);

== matlab function feedbacklin/Output ==
  data: x input; y output
function y = output(x)

% Output(3x1)
y = zeros(3,1);
y(1) = x(1);
y(2) = x(2);
y(3) = x(7);

% y = [x(1), x(2), 0, 0, 0, 0, x(7), 0, 0, 0, 0, 0];
